simulink model "carrierbased"  (R2015b)
settings: Solver=VariableStepAuto  StartTime=0.0  StopTime=10  RelTol=1e-3
libraries: powerlib x33, simulink x6, powerlib_meascontrol x2
settings Model: Creator=hakan  LastModifiedBy=hakan

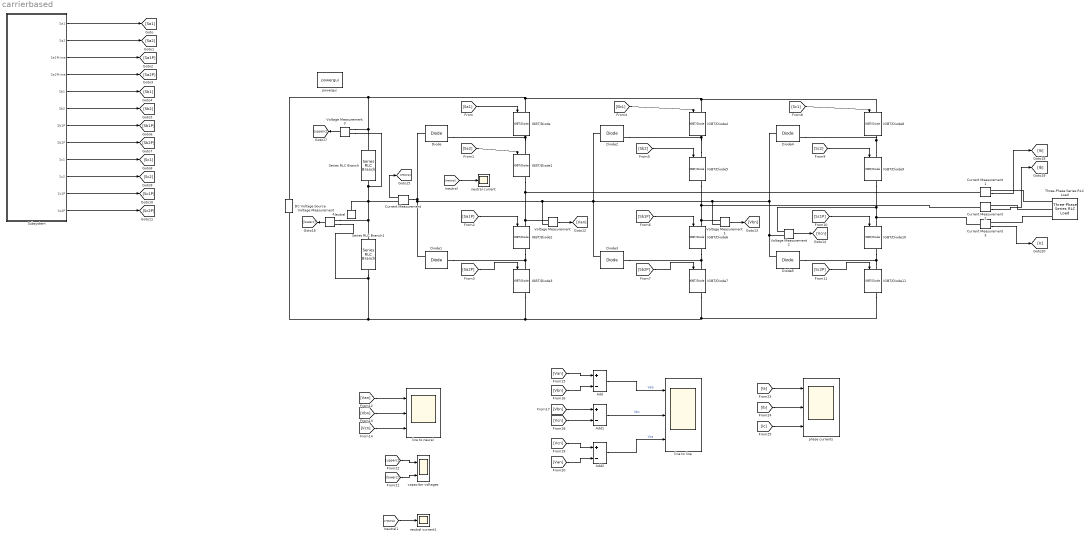
== system carrierbased ==
  Add : Sum  Inputs=+-
  Add1 : Sum  Inputs=+-
  Add2 : Sum  Inputs=+-
  Current Measurement{,1..3} (4 alike) : powerlib/Measurements/Current Measurement  PhasorSimulation=off  OutputType=Complex  PSBequivalent=0
  DC Voltage Source : powerlib/Electrical Sources/DC Voltage Source  Amplitude=540  Measurements=None
  Diode{,1..5} (6 alike) : powerlib/Power Electronics/Diode  Ron=0.001  Lon=0  Vf=0.8  IC=0  UseSnubber=off  Rs=500  Cs=250e-9  Measurements=on
  IGBT/Diode{,1..11} (12 alike) : powerlib/Power Electronics/IGBT//Diode  Ron=1e-3  Rs=1e5  Cs=inf  Measurements=on
  Neutral : powerlib/Elements/Neutral  LConnTagsString=a  NodeNumber=10
  Series RLC Branch : powerlib/Elements/Series RLC Branch  LConnTagsString=__new0  RConnTagsString=__new0  BranchType=RC  Resistance=1  Inductance=1e-3  SetiL0=off  InitialCurrent=0  Capacitance=1000e-6  Setx0=off  InitialVoltage=0  Measurements=None
  Series RLC Branch1 : powerlib/Elements/Series RLC Branch  LConnTagsString=__new0  RConnTagsString=__new0  BranchType=RC  Resistance=1  Inductance=1e-3  SetiL0=off  InitialCurrent=0  Capacitance=1000e-6  Setx0=off  InitialVoltage=0  Measurements=None
  Subsystem : Subsystem
  Three-Phase Series RLC Load : powerlib/Elements/Three-Phase Series RLC Load  LConnTagsString=A|B|C  Configuration=Y (grounded)  NominalVoltage=1000  Vabc=[1e3 1e3 1e3]  Vabcp=[1e3 1e3 1e3]  NominalFrequency=50  UnbalancedPower=off  ActivePower=8000  InductivePower=3870  CapacitivePower=0  Pabc=[10e3 9e3 11e3]  QLabc=[100 90 110]  QCabc=[100 90 110]  Pabcp=[10e3 9e3 11e3]  QLabcp=[100 90 110]  QCabcp=[100 90 110]  Measurements=None  LoadType=constant Z
  Voltage Measurement{,1..4} (5 alike) : powerlib/Measurements/Voltage Measurement  PhasorSimulation=off  OutputType=Complex  PSBequivalent=0
  capacitor voltages : Scope  NumInputPorts=2
  line to line : Scope  NumInputPorts=3
  line to neural : Scope  NumInputPorts=3
  neutral current : Scope
  neutral current1 : Scope
  phase currents : Scope  NumInputPorts=3
  powergui : powerlib/powergui  Priority=1  SimulationMode=Continuous  SolverType=Tustin/Backward Euler (TBE)  SampleTime=50e-6  frequency=60  SPID=off  DisableSnubberDevices=off  DisableRonSwitches=off  DisableVfSwitches=off  SwTol=0  DisplayEquations=off  Interpol=off  ExternalGateDelay=off  methode=off  Ts=10  FunctionMessages=off  echomessages=off  HookPort=off  EnableUseOfTLC=off  x0status=blocks  frequencyindice=0  Pbase=100e6  ErrMax=1e-4  Iterations=50  UnitsV=kV  UnitsW=MW  buscounter=0  RestoreLinks=warning  ResistiveCurrentMeasurement=off  Frange=[0:2:500]  Ylog=off  Xlog=on  ShowGrid=off  save=off  variable=ZData  structure=0  ZoomFFT=off  StartTime=0.0  cycles=1  DisplayStyle=1  fundamental=60  FreqAxis=off  MaxFrequency=1000  frequencyindicesteady=1  RmsSteady=1  display=off
  wires:
  Subsystem/1("Sa1 ") -> [Sa1]
  Subsystem/2("Sa2 ") -> [Sa2]
  Subsystem/3(Sa1Prime) -> [Sa1P]
  Subsystem/4("Sa2Prime ") -> [Sa2P]
  [Sa1] -> IGBT/Diode/1
  [Sa2] -> IGBT/Diode1/1
  [Sa1P] -> IGBT/Diode2/1
  [Sa2P] -> IGBT/Diode3/1
  [Sb1] -> IGBT/Diode4/1
  [Sb2] -> IGBT/Diode5/1
  [Sb1P] -> IGBT/Diode6/1
  [Sb2P] -> IGBT/Diode7/1
  [Sc1] -> IGBT/Diode8/1
  [Sc2] -> IGBT/Diode9/1
  [Sc1P] -> IGBT/Diode10/1
  [Sc2P] -> IGBT/Diode11/1
  Voltage Measurement/1 -> [Van]
  Subsystem/5(Sb1) -> [Sb1]
  Subsystem/6(Sb2) -> [Sb2]
  Subsystem/7("Sb1P ") -> [Sb1P]
  Subsystem/8(Sb2P) -> [Sb2P]
  Subsystem/9("Sc1 ") -> [Sc1]
  Subsystem/10(Sc2) -> [Sc2]
  Subsystem/11(Sc1P) -> [Sc1P]
  Subsystem/12("Sc2P ") -> [Sc2P]
  Voltage Measurement1/1 -> [Vbn]
  Voltage Measurement2/1 -> [Vcn]
  [Van] -> Add/1
  [Vbn] -> Add/2
  Add/1 -> line to line/1  "Vab"
  [Vbn] -> Add1/1
  [Vcn] -> Add1/2
  Add1/1 -> line to line/2  "Vbc"
  [Vcn] -> Add2/1
  [Van] -> Add2/2
  Add2/1 -> line to line/3  "Vca"
  [Van] -> line to neural/1
  [Vbn] -> line to neural/2
  [Vcn] -> line to neural/3
  Voltage Measurement3/1 -> [upperc]
  Voltage Measurement4/1 -> [lowerc]
  [lowerc] -> capacitor voltages/2
  [upperc] -> capacitor voltages/1
  Current Measurement/1 -> [Ineutral]
  [Ineutral] -> neutral current/1
  [Ineutral] -> neutral current1/1
  Current Measurement1/1 -> [Ia]
  Current Measurement2/1 -> [Ib]
  Current Measurement3/1 -> [Ic]
  [Ib] -> phase currents/2
  [Ia] -> phase currents/1
  [Ic] -> phase currents/3
  connections:
  DC Voltage Source/RConn1 -- IGBT/Diode8/LConn1 -- IGBT/Diode4/LConn1 -- IGBT/Diode/LConn1 -- Series RLC Branch/LConn1 -- Voltage Measurement3/LConn1
  Series RLC Branch1/RConn1 -- Voltage Measurement4/LConn2 -- IGBT/Diode11/RConn1 -- IGBT/Diode7/RConn1 -- IGBT/Diode3/RConn1 -- DC Voltage Source/LConn1
  IGBT/Diode/RConn1 -- IGBT/Diode1/LConn1 -- Diode/RConn1
  IGBT/Diode1/RConn1 -- Voltage Measurement/LConn1 -- IGBT/Diode2/LConn1 -- Current Measurement1/LConn1
  IGBT/Diode2/RConn1 -- Diode1/LConn1 -- IGBT/Diode3/LConn1
  Diode5/RConn1 -- Diode4/LConn1 -- Voltage Measurement1/LConn2 -- Diode3/RConn1 -- Voltage Measurement/LConn2 -- Diode/LConn1 -- Current Measurement/LConn1 -- Diode1/RConn1 -- Diode2/LConn1 -- Voltage Measurement2/LConn2
  IGBT/Diode5/LConn1 -- Diode2/RConn1 -- IGBT/Diode4/RConn1
  IGBT/Diode6/RConn1 -- Diode3/LConn1 -- IGBT/Diode7/LConn1
  IGBT/Diode5/RConn1 -- Voltage Measurement1/LConn1 -- IGBT/Diode6/LConn1 -- Current Measurement2/LConn1
  Diode4/RConn1 -- IGBT/Diode8/RConn1 -- IGBT/Diode9/LConn1
  Diode5/LConn1 -- IGBT/Diode11/LConn1 -- IGBT/Diode10/RConn1
  IGBT/Diode9/RConn1 -- Voltage Measurement2/LConn1 -- IGBT/Diode10/LConn1 -- Current Measurement3/LConn1
  Series RLC Branch/RConn1 -- Voltage Measurement3/LConn2 -- Current Measurement/RConn1 -- Neutral/LConn1 -- Voltage Measurement4/LConn1 -- Series RLC Branch1/LConn1
  Three-Phase Series RLC Load/LConn3 -- Current Measurement3/RConn1
  Three-Phase Series RLC Load/LConn2 -- Current Measurement2/RConn1
  Three-Phase Series RLC Load/LConn1 -- Current Measurement1/RConn1

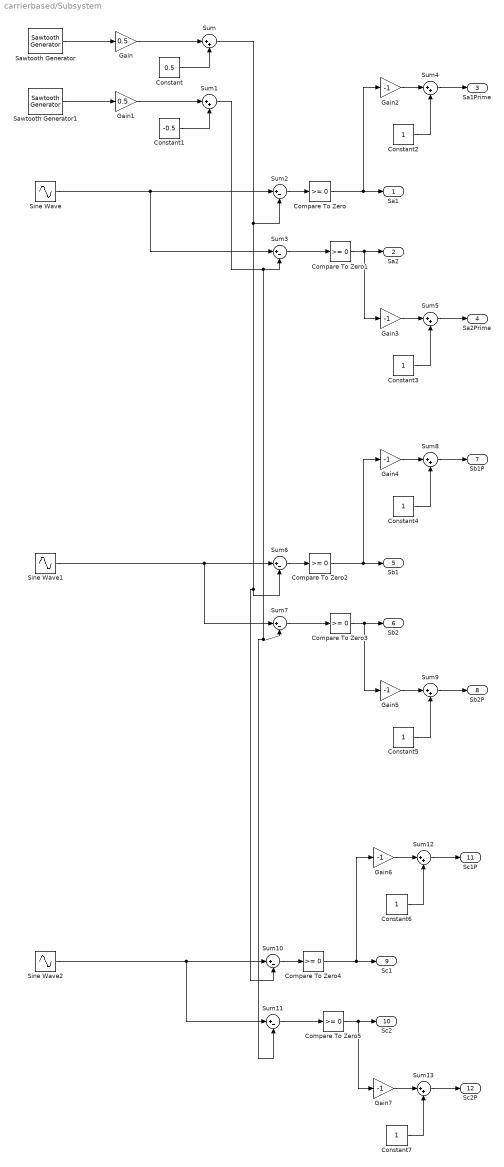
== system carrierbased/Subsystem ==
  Compare To Zero{,1..5} (6 alike) : simulink/Logic and Bit Operations/Compare To Zero  relop=>=  OutDataTypeStr=boolean
  Constant : Constant  Value=0.5
  Constant1 : Constant  Value=-0.5
  Constant{2..7} (6 alike) : Constant
  Gain : Gain  Gain=0.5
  Gain1 : Gain  Gain=0.5
  Gain{2..7} (6 alike) : Gain  Gain=-1
  Sawtooth Generator : powerlib_meascontrol/Pulse & Signal Generators/Sawtooth Generator  Freq=2e3  Phase=180  Ts=0
  Sawtooth Generator1 : powerlib_meascontrol/Pulse & Signal Generators/Sawtooth Generator  Freq=2e3  Phase=180  Ts=0
  Sine Wave : Sin  Amplitude=0.8  Frequency=100*pi  SampleTime=0
  Sine Wave1 : Sin  Amplitude=0.8  Frequency=100*pi  Phase=2*pi/3  SampleTime=0
  Sine Wave2 : Sin  Amplitude=0.8  Frequency=100*pi  Phase=4*pi/3  SampleTime=0
  Sum{,1,4..5,8..9,12..13} (8 alike) : Sum  Inputs=|++
  Sum{2..3,6..7,10..11} (6 alike) : Sum  Inputs=|+-
  "Sa1 " : Outport
  "Sa2 " : Outport  Port=2
  Sa1Prime : Outport  Port=3
  "Sa2Prime " : Outport  Port=4
  Sb1 : Outport  Port=5
  Sb2 : Outport  Port=6
  "Sb1P " : Outport  Port=7
  Sb2P : Outport  Port=8
  "Sc1 " : Outport  Port=9
  Sc2 : Outport  Port=10
  Sc1P : Outport  Port=11
  "Sc2P " : Outport  Port=12
  wires:
  Sawtooth Generator/1 -> Gain/1
  Gain/1 -> Sum/1
  Sum/1 -> Sum2/2, Sum10/2, Sum6/2
  Constant/1 -> Sum/2
  Sawtooth Generator1/1 -> Gain1/1
  Gain1/1 -> Sum1/1
  Sum1/1 -> Sum11/2, Sum7/2, Sum3/2
  Constant1/1 -> Sum1/2
  Sine Wave/1 -> Sum3/1, Sum2/1
  Sum2/1 -> Compare To Zero/1
  Compare To Zero/1 -> Gain2/1, "Sa1 "/1
  Sum3/1 -> Compare To Zero1/1
  Compare To Zero1/1 -> Gain3/1, "Sa2 "/1
  Constant2/1 -> Sum4/2
  Gain2/1 -> Sum4/1
  Sum4/1 -> Sa1Prime/1
  Constant3/1 -> Sum5/2
  Gain3/1 -> Sum5/1
  Sum5/1 -> "Sa2Prime "/1
  Sum6/1 -> Compare To Zero2/1
  Compare To Zero2/1 -> Sb1/1, Gain4/1
  Sum7/1 -> Compare To Zero3/1
  Compare To Zero3/1 -> Sb2/1, Gain5/1
  Constant4/1 -> Sum8/2
  Gain4/1 -> Sum8/1
  Sum8/1 -> "Sb1P "/1
  Constant5/1 -> Sum9/2
  Gain5/1 -> Sum9/1
  Sum9/1 -> Sb2P/1
  Sine Wave1/1 -> Sum7/1, Sum6/1
  Sum10/1 -> Compare To Zero4/1
  Compare To Zero4/1 -> Gain6/1, "Sc1 "/1
  Sum11/1 -> Compare To Zero5/1
  Compare To Zero5/1 -> Gain7/1, Sc2/1
  Constant6/1 -> Sum12/2
  Gain6/1 -> Sum12/1
  Sum12/1 -> Sc1P/1
  Constant7/1 -> Sum13/2
  Gain7/1 -> Sum13/1
  Sum13/1 -> "Sc2P "/1
  Sine Wave2/1 -> Sum11/1, Sum10/1
